simulink model "MPC_RL_H2DF"  (R2023a)
settings: Solver=FixedStepAuto  StartTime=0.0  StopTime=inf  FixedStep=Ts  RelTol=1e-3
model workspace (MAT data in the model file):
  enable_IMEP_noise = 100
  enable_IMEP_offset = 1
values from neighbouring files (symbols this model uses):
  C2C_NMPC = init_C2C_NMPC_H2DF(C2C_NMPC.expdata)    [init_H2DFRL_GRU.m]
  LowerLimit = ([0.17e-3;350;-5;1e-3] - C2C_NMPC.Normalization.controls.mean)./(C2C_NMPC.Normalization.controls.std)    [init_H2DFRL_GRU.m]
  Ts = 0.08    [init_H2DFRL_GRU.m]
  UpperLimit = ([0.5e-3;900;2;5.5e-3] - C2C_NMPC.Normalization.controls.mean)./(C2C_NMPC.Normalization.controls.std)    [init_H2DFRL_GRU.m]
undefined symbols (not defined in the file or in its folder): CA50_offset, DiscIntNeverNeededParam, enable_CA50_noise, enable_CA50_offset, IMEP_offset
libraries: simulink x15, matrix_library x6, dspsigattribs x2, slctrlblks x2, statsLibrary x1, rllib x1
(part 4 of 4)

== system MPC_RL_H2DF/Engine Model2/C2C_NMPC_n2/constraints/Normalizing data ==
  physical_data : Inport
  Constant1 : Constant  Value=C2C_NMPC.Normalization.controls.mean(2)
  Constant2 : Constant  Value=C2C_NMPC.Normalization.controls.mean(3)
  Constant3 : Constant  Value=C2C_NMPC.Normalization.controls.mean(1)
  Constant4 : Constant  Value=C2C_NMPC.Normalization.controls.mean(4)
  Gain1 : Gain  Gain=1/C2C_NMPC.Normalization.controls.std(2)
  Gain2 : Gain  Gain=1/C2C_NMPC.Normalization.controls.std(3)
  Gain3 : Gain  Gain=1/C2C_NMPC.Normalization.controls.std(4)
  Gain4 : Gain  Gain=1/C2C_NMPC.Normalization.controls.std(1)
  Mux : Mux
  Selector : Selector  IndexOptions=Index vector (dialog)  Indices=[2]  OutputSizes=1
  Selector1 : Selector  IndexOptions=Index vector (dialog)  Indices=[1]  OutputSizes=1
  Selector2 : Selector  IndexOptions=Index vector (dialog)  Indices=[3]  OutputSizes=1
  Selector3 : Selector  IndexOptions=Index vector (dialog)  Indices=[4]  OutputSizes=1
  Sum{1..4} (4 alike) : Sum  Inputs=|+-
  normalized_data : Outport
  wires:
  Constant3/1 -> Sum4/2
  Selector2/1 -> Sum3/1
  Constant2/1 -> Sum3/2
  Sum4/1 -> Gain4/1
  Sum3/1 -> Gain2/1
  Selector/1 -> Sum2/1
  Constant1/1 -> Sum2/2
  Sum2/1 -> Gain1/1
  Sum1/1 -> Gain3/1
  Constant4/1 -> Sum1/2
  Selector3/1 -> Sum1/1
  Selector1/1 -> Sum4/1
  Gain4/1 -> Mux/1
  Gain1/1 -> Mux/2
  Gain2/1 -> Mux/3
  Gain3/1 -> Mux/4
  Mux/1 -> normalized_data/1
  physical_data/1 -> Selector1/1, Selector/1, Selector3/1, Selector2/1

== system MPC_RL_H2DF/Engine Model2/C2C_NMPC_n2/constraints/Normalizing data1 ==
  physical_data : Inport
  Constant1 : Constant  Value=C2C_NMPC.Normalization.controls.mean(2)
  Constant2 : Constant  Value=C2C_NMPC.Normalization.controls.mean(3)
  Constant3 : Constant  Value=C2C_NMPC.Normalization.controls.mean(1)
  Constant4 : Constant  Value=C2C_NMPC.Normalization.controls.mean(4)
  Gain1 : Gain  Gain=1/C2C_NMPC.Normalization.controls.std(2)
  Gain2 : Gain  Gain=1/C2C_NMPC.Normalization.controls.std(3)
  Gain3 : Gain  Gain=1/C2C_NMPC.Normalization.controls.std(4)
  Gain4 : Gain  Gain=1/C2C_NMPC.Normalization.controls.std(1)
  Mux : Mux
  Selector : Selector  IndexOptions=Index vector (dialog)  Indices=[2]  OutputSizes=1
  Selector1 : Selector  IndexOptions=Index vector (dialog)  Indices=[1]  OutputSizes=1
  Selector2 : Selector  IndexOptions=Index vector (dialog)  Indices=[3]  OutputSizes=1
  Selector3 : Selector  IndexOptions=Index vector (dialog)  Indices=[4]  OutputSizes=1
  Sum{1..4} (4 alike) : Sum  Inputs=|+-
  normalized_data : Outport
  wires:
  Constant3/1 -> Sum4/2
  Selector2/1 -> Sum3/1
  Constant2/1 -> Sum3/2
  Sum4/1 -> Gain4/1
  Sum3/1 -> Gain2/1
  Selector/1 -> Sum2/1
  Constant1/1 -> Sum2/2
  Sum2/1 -> Gain1/1
  Sum1/1 -> Gain3/1
  Constant4/1 -> Sum1/2
  Selector3/1 -> Sum1/1
  Selector1/1 -> Sum4/1
  Gain4/1 -> Mux/1
  Gain1/1 -> Mux/2
  Gain2/1 -> Mux/3
  Gain3/1 -> Mux/4
  Mux/1 -> normalized_data/1
  physical_data/1 -> Selector1/1, Selector/1, Selector3/1, Selector2/1

== system MPC_RL_H2DF/Engine Model2/C2C_NMPC_n2/constraints/Subsystem ==
  In : Inport
  Constant : Constant  Value=C2C_NMPC.Normalization.outputs.mean(1)
  Constant1 : Constant  Value=C2C_NMPC.Normalization.outputs.mean(2)
  Constant2 : Constant  Value=C2C_NMPC.Normalization.outputs.mean(3)
  Constant3 : Constant  Value=C2C_NMPC.Normalization.outputs.mean(4)
  Demux : Demux
  Gain : Gain  Gain=1/C2C_NMPC.Normalization.outputs.std(1)
  Gain1 : Gain  Gain=1/C2C_NMPC.Normalization.outputs.std(2)
  Gain2 : Gain  Gain=1/C2C_NMPC.Normalization.outputs.std(3)
  Gain3 : Gain  Gain=1/C2C_NMPC.Normalization.outputs.std(4)
  Mux : Mux
  Sum{1..3,5} (4 alike) : Sum  Inputs=|+-
  value : Outport
  wires:
  Constant/1 -> Sum5/2
  Constant1/1 -> Sum1/2
  Sum1/1 -> Gain1/1
  Demux/3 -> Sum2/1
  Sum2/1 -> Gain2/1
  Constant2/1 -> Sum2/2
  Gain/1 -> Mux/1
  Sum3/1 -> Gain3/1
  Constant3/1 -> Sum3/2
  Sum5/1 -> Gain/1
  Demux/1 -> Sum5/1
  Gain2/1 -> Mux/3
  Gain3/1 -> Mux/4
  Gain1/1 -> Mux/2
  Demux/2 -> Sum1/1
  Demux/4 -> Sum3/1
  In/1 -> Demux/1
  Mux/1 -> value/1

== system MPC_RL_H2DF/Engine Model2/C2C_NMPC_n2/constraints/Subsystem1 ==
  In : Inport
  Constant : Constant  Value=C2C_NMPC.Normalization.outputs.mean(1)
  Constant1 : Constant  Value=C2C_NMPC.Normalization.outputs.mean(2)
  Constant2 : Constant  Value=C2C_NMPC.Normalization.outputs.mean(3)
  Constant3 : Constant  Value=C2C_NMPC.Normalization.outputs.mean(4)
  Demux : Demux
  Gain : Gain  Gain=1/C2C_NMPC.Normalization.outputs.std(1)
  Gain1 : Gain  Gain=1/C2C_NMPC.Normalization.outputs.std(2)
  Gain2 : Gain  Gain=1/C2C_NMPC.Normalization.outputs.std(3)
  Gain3 : Gain  Gain=1/C2C_NMPC.Normalization.outputs.std(4)
  Mux : Mux
  Sum{1..3,5} (4 alike) : Sum  Inputs=|+-
  ubh_e : Outport
  wires:
  Mux/1 -> ubh_e/1
  In/1 -> Demux/1
  Demux/4 -> Sum3/1
  Demux/2 -> Sum1/1
  Gain1/1 -> Mux/2
  Gain3/1 -> Mux/4
  Gain2/1 -> Mux/3
  Demux/1 -> Sum5/1
  Sum5/1 -> Gain/1
  Constant3/1 -> Sum3/2
  Sum3/1 -> Gain3/1
  Gain/1 -> Mux/1
  Constant2/1 -> Sum2/2
  Sum2/1 -> Gain2/1
  Demux/3 -> Sum2/1
  Sum1/1 -> Gain1/1
  Constant1/1 -> Sum1/2
  Constant/1 -> Sum5/2

== system MPC_RL_H2DF/Engine Model2/C2C_NMPC_n2/constraints/Subsystem2 ==
  In : Inport
  Demux : Demux
  Gain : Gain  Gain=1/C2C_NMPC.Normalization.controls.std(1)
  Gain1 : Gain  Gain=1/C2C_NMPC.Normalization.controls.std(2)
  Gain2 : Gain  Gain=1/C2C_NMPC.Normalization.controls.std(3)
  Gain3 : Gain  Gain=1/C2C_NMPC.Normalization.controls.std(4)
  Mux : Mux
  Out : Outport
  wires:
  Gain/1 -> Mux/1
  Gain2/1 -> Mux/3
  Gain1/1 -> Mux/2
  In/1 -> Demux/1
  Mux/1 -> Out/1
  Demux/1 -> Gain/1
  Demux/2 -> Gain1/1
  Demux/3 -> Gain2/1
  Demux/4 -> Gain3/1
  Gain3/1 -> Mux/4

== system MPC_RL_H2DF/Engine Model2/C2C_NMPC_n2/constraints/Subsystem3 ==
  In : Inport
  Demux : Demux
  Gain : Gain  Gain=1/C2C_NMPC.Normalization.controls.std(1)
  Gain1 : Gain  Gain=1/C2C_NMPC.Normalization.controls.std(2)
  Gain2 : Gain  Gain=1/C2C_NMPC.Normalization.controls.std(3)
  Gain3 : Gain  Gain=1/C2C_NMPC.Normalization.controls.std(4)
  Mux : Mux
  Out : Outport
  wires:
  Gain/1 -> Mux/1
  Gain2/1 -> Mux/3
  Gain1/1 -> Mux/2
  In/1 -> Demux/1
  Mux/1 -> Out/1
  Demux/1 -> Gain/1
  Demux/2 -> Gain1/1
  Demux/3 -> Gain2/1
  Demux/4 -> Gain3/1
  Gain3/1 -> Mux/4

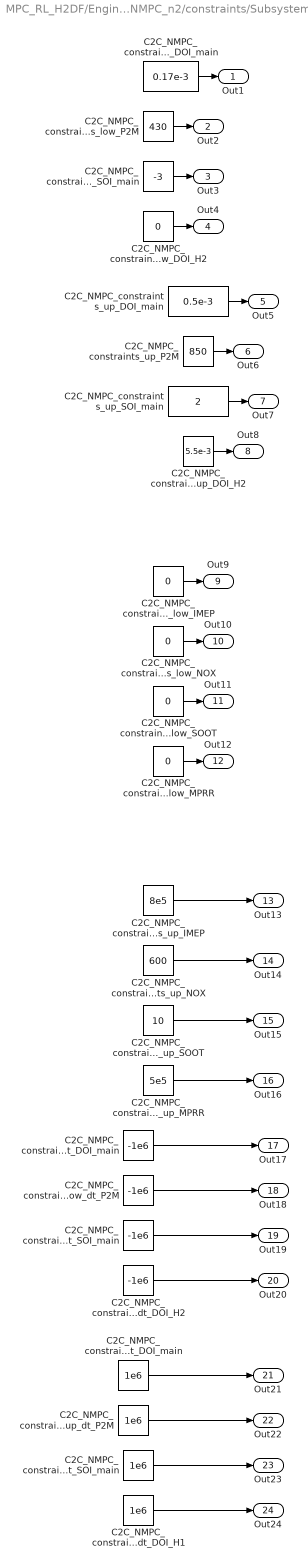
== system MPC_RL_H2DF/Engine Model2/C2C_NMPC_n2/constraints/Subsystem4 ==
  C2C_NMPC_constraints_low_DOI_H2 : Constant  Value=0
  C2C_NMPC_constraints_low_DOI_main : Constant  Value=0.17e-3
  C2C_NMPC_constraints_low_IMEP : Constant  Value=0
  C2C_NMPC_constraints_low_MPRR : Constant  Value=0
  C2C_NMPC_constraints_low_NOX : Constant  Value=0
  C2C_NMPC_constraints_low_P2M : Constant  Value=430
  C2C_NMPC_constraints_low_SOI_main : Constant  Value=-3
  C2C_NMPC_constraints_low_SOOT : Constant  Value=0
  C2C_NMPC_constraints_low_dt_DOI_H2 : Constant  Value=-1e6
  C2C_NMPC_constraints_low_dt_DOI_main : Constant  Value=-1e6
  C2C_NMPC_constraints_low_dt_P2M : Constant  Value=-1e6
  C2C_NMPC_constraints_low_dt_SOI_main : Constant  Value=-1e6
  C2C_NMPC_constraints_up_DOI_H2 : Constant  Value=5.5e-3
  C2C_NMPC_constraints_up_DOI_main : Constant  Value=0.5e-3
  C2C_NMPC_constraints_up_IMEP : Constant  Value=8e5
  C2C_NMPC_constraints_up_MPRR : Constant  Value=5e5
  C2C_NMPC_constraints_up_NOX : Constant  Value=600
  C2C_NMPC_constraints_up_P2M : Constant  Value=850
  C2C_NMPC_constraints_up_SOI_main : Constant  Value=2
  C2C_NMPC_constraints_up_SOOT : Constant  Value=10
  C2C_NMPC_constraints_up_dt_DOI_H1 : Constant  Value=1e6
  C2C_NMPC_constraints_up_dt_DOI_main : Constant  Value=1e6
  C2C_NMPC_constraints_up_dt_P2M : Constant  Value=1e6
  C2C_NMPC_constraints_up_dt_SOI_main : Constant  Value=1e6
  Out1 : Outport
  Out2 : Outport  Port=2
  Out3 : Outport  Port=3
  Out4 : Outport  Port=4
  Out5 : Outport  Port=5
  Out6 : Outport  Port=6
  Out7 : Outport  Port=7
  Out8 : Outport  Port=8
  Out9 : Outport  Port=9
  Out10 : Outport  Port=10
  Out11 : Outport  Port=11
  Out12 : Outport  Port=12
  Out13 : Outport  Port=13
  Out14 : Outport  Port=14
  Out15 : Outport  Port=15
  Out16 : Outport  Port=16
  Out17 : Outport  Port=17
  Out18 : Outport  Port=18
  Out19 : Outport  Port=19
  Out20 : Outport  Port=20
  Out21 : Outport  Port=21
  Out22 : Outport  Port=22
  Out23 : Outport  Port=23
  Out24 : Outport  Port=24
  wires:
  C2C_NMPC_constraints_low_dt_DOI_H2/1 -> Out20/1
  C2C_NMPC_constraints_low_dt_P2M/1 -> Out18/1
  C2C_NMPC_constraints_up_dt_SOI_main/1 -> Out23/1
  C2C_NMPC_constraints_up_dt_DOI_H1/1 -> Out24/1
  C2C_NMPC_constraints_up_DOI_H2/1 -> Out8/1
  C2C_NMPC_constraints_low_dt_DOI_main/1 -> Out17/1
  C2C_NMPC_constraints_low_dt_SOI_main/1 -> Out19/1
  C2C_NMPC_constraints_up_SOOT/1 -> Out15/1
  C2C_NMPC_constraints_up_MPRR/1 -> Out16/1
  C2C_NMPC_constraints_up_NOX/1 -> Out14/1
  C2C_NMPC_constraints_up_IMEP/1 -> Out13/1
  C2C_NMPC_constraints_up_dt_P2M/1 -> Out22/1
  C2C_NMPC_constraints_low_SOI_main/1 -> Out3/1
  C2C_NMPC_constraints_up_dt_DOI_main/1 -> Out21/1
  C2C_NMPC_constraints_low_SOOT/1 -> Out11/1
  C2C_NMPC_constraints_low_DOI_H2/1 -> Out4/1
  C2C_NMPC_constraints_up_P2M/1 -> Out6/1
  C2C_NMPC_constraints_low_P2M/1 -> Out2/1
  C2C_NMPC_constraints_low_DOI_main/1 -> Out1/1
  C2C_NMPC_constraints_low_MPRR/1 -> Out12/1
  C2C_NMPC_constraints_up_SOI_main/1 -> Out7/1
  C2C_NMPC_constraints_up_DOI_main/1 -> Out5/1
  C2C_NMPC_constraints_low_IMEP/1 -> Out9/1
  C2C_NMPC_constraints_low_NOX/1 -> Out10/1

== system MPC_RL_H2DF/Engine Model2/C2C_NMPC_n2/cost_function_weights/Normalize 0 to 1 ==
  In1 : Inport
  Demux : Demux
  Divide{,1..3} (4 alike) : Product  Inputs=*/
  Mux : Mux
  Sum : Sum  Inputs=|++++
  Out1 : Outport
  wires:
  In1/1 -> Demux/1
  Demux/1 -> Sum/1, Divide/1
  Demux/2 -> Divide1/1, Sum/2
  Demux/3 -> Divide2/1, Sum/3
  Demux/4 -> Divide3/1, Sum/4
  Sum/1 -> Divide/2, Divide1/2, Divide2/2, Divide3/2
  Divide3/1 -> Mux/4
  Divide2/1 -> Mux/3
  Divide1/1 -> Mux/2
  Divide/1 -> Mux/1
  Mux/1 -> Out1/1

== system MPC_RL_H2DF/Engine Model2/offset_and_noise/CA50_generation/denormalizing_CA50 ==
  CA50_in : Inport
  Constant : Constant  Value=C2C_NMPC.Normalization.outputs.mean(4)
  Gain : Gain  Gain=C2C_NMPC.Normalization.outputs.std(4)
  Sum5 : Sum  Inputs=|++
  CA50 : Outport
  wires:
  CA50_in/1 -> Gain/1
  Gain/1 -> Sum5/1
  Constant/1 -> Sum5/2
  Sum5/1 -> CA50/1

== system MPC_RL_H2DF/Engine Model2/offset_and_noise/CA50_generation/normalizing_CA50 ==
  CA50 : Inport
  Constant : Constant  Value=C2C_NMPC.Normalization.outputs.mean(4)
  Gain : Gain  Gain=1/C2C_NMPC.Normalization.outputs.std(4)
  Sum5 : Sum  Inputs=|+-
  CA50_out : Outport
  wires:
  CA50/1 -> Sum5/1
  Constant/1 -> Sum5/2
  Gain/1 -> CA50_out/1
  Sum5/1 -> Gain/1

== system MPC_RL_H2DF/Engine Model2/offset_and_noise/IMEP_generation/denormalizing_IMEP ==
  IMEP_in : Inport
  Constant : Constant  Value=C2C_NMPC.Normalization.outputs.mean(1)
  Gain : Gain  Gain=C2C_NMPC.Normalization.outputs.std(1)
  Sum5 : Sum  Inputs=|++
  IMEP : Outport
  wires:
  IMEP_in/1 -> Gain/1
  Gain/1 -> Sum5/1
  Constant/1 -> Sum5/2
  Sum5/1 -> IMEP/1

== system MPC_RL_H2DF/Engine Model2/offset_and_noise/IMEP_generation/normalizing_IMEP ==
  IMEP : Inport
  Constant : Constant  Value=C2C_NMPC.Normalization.outputs.mean(1)
  Gain : Gain  Gain=1/C2C_NMPC.Normalization.outputs.std(1)
  Sum5 : Sum  Inputs=|+-
  IMEP_out : Outport
  wires:
  IMEP/1 -> Sum5/1
  Constant/1 -> Sum5/2
  Gain/1 -> IMEP_out/1
  Sum5/1 -> Gain/1

== system MPC_RL_H2DF/Engine Model2/offset_and_noise1/IMEP_generation/denormalizing_IMEP ==
  IMEP_in : Inport
  Constant : Constant  Value=C2C_NMPC.Normalization.outputs.mean(1)
  Gain : Gain  Gain=C2C_NMPC.Normalization.outputs.std(1)
  Sum5 : Sum  Inputs=|++
  IMEP : Outport
  wires:
  IMEP_in/1 -> Gain/1
  Gain/1 -> Sum5/1
  Constant/1 -> Sum5/2
  Sum5/1 -> IMEP/1

== system MPC_RL_H2DF/Engine Model2/offset_and_noise1/IMEP_generation/normalizing_IMEP ==
  IMEP : Inport
  Constant : Constant  Value=C2C_NMPC.Normalization.outputs.mean(1)
  Gain : Gain  Gain=1/C2C_NMPC.Normalization.outputs.std(1)
  Sum5 : Sum  Inputs=|+-
  IMEP_out : Outport
  wires:
  IMEP/1 -> Sum5/1
  Constant/1 -> Sum5/2
  Gain/1 -> IMEP_out/1
  Sum5/1 -> Gain/1

== system MPC_RL_H2DF/Engine Model2/offset_and_noise2/IMEP_generation/denormalizing_IMEP ==
  IMEP_in : Inport
  Constant : Constant  Value=C2C_NMPC.Normalization.outputs.mean(1)
  Gain : Gain  Gain=C2C_NMPC.Normalization.outputs.std(1)
  Sum5 : Sum  Inputs=|++
  IMEP : Outport
  wires:
  IMEP_in/1 -> Gain/1
  Gain/1 -> Sum5/1
  Constant/1 -> Sum5/2
  Sum5/1 -> IMEP/1

== system MPC_RL_H2DF/Engine Model2/offset_and_noise2/IMEP_generation/normalizing_IMEP ==
  IMEP : Inport
  Constant : Constant  Value=C2C_NMPC.Normalization.outputs.mean(1)
  Gain : Gain  Gain=1/C2C_NMPC.Normalization.outputs.std(1)
  Sum5 : Sum  Inputs=|+-
  IMEP_out : Outport
  wires:
  IMEP/1 -> Sum5/1
  Constant/1 -> Sum5/2
  Gain/1 -> IMEP_out/1
  Sum5/1 -> Gain/1

== system MPC_RL_H2DF/Engine Model2/offset_and_noise3/IMEP_generation/denormalizing_IMEP ==
  IMEP_in : Inport
  Constant : Constant  Value=C2C_NMPC.Normalization.outputs.mean(1)
  Gain : Gain  Gain=C2C_NMPC.Normalization.outputs.std(1)
  Sum5 : Sum  Inputs=|++
  IMEP : Outport
  wires:
  IMEP_in/1 -> Gain/1
  Gain/1 -> Sum5/1
  Constant/1 -> Sum5/2
  Sum5/1 -> IMEP/1

== system MPC_RL_H2DF/Engine Model2/offset_and_noise3/IMEP_generation/normalizing_IMEP ==
  IMEP : Inport
  Constant : Constant  Value=C2C_NMPC.Normalization.outputs.mean(1)
  Gain : Gain  Gain=1/C2C_NMPC.Normalization.outputs.std(1)
  Sum5 : Sum  Inputs=|+-
  IMEP_out : Outport
  wires:
  IMEP/1 -> Sum5/1
  Constant/1 -> Sum5/2
  Gain/1 -> IMEP_out/1
  Sum5/1 -> Gain/1

== system MPC_RL_H2DF/Signal Processing/calculate reward/Subsystem/ControlError ==
  ReferenceControls : Inport
  Controls : Inport  Port=2
  Demux1 : Demux
  Demux2 : Demux
  Mux : Mux
  Subtract{,1..3} (4 alike) : Sum  Inputs=+-
  ControlError : Outport
  wires:
  Demux2/4 -> Subtract3/2
  Demux1/2 -> Subtract1/1
  Demux1/1 -> Subtract/1
  Demux2/2 -> Subtract1/2
  Demux2/3 -> Subtract2/2
  Controls/1 -> Demux2/1
  Demux1/3 -> Subtract2/1
  Demux1/4 -> Subtract3/1
  Demux2/1 -> Subtract/2
  Mux/1 -> ControlError/1
  Subtract/1 -> Mux/1
  Subtract1/1 -> Mux/2
  Subtract2/1 -> Mux/3
  Subtract3/1 -> Mux/4
  ReferenceControls/1 -> Demux1/1

== system MPC_RL_H2DF/Signal Processing/calculate reward/Subsystem/Staging ==
  Output : Inport
  Reference_Output : Inport  Port=2
  Abs4 : Abs  SaturateOnIntegerOverflow=off
  Add : Sum  Inputs=++++
  Constant : Constant  Value=100000
  Constant1 : Constant  Value=10000
  Constant2 : Constant  Value=1000
  Constant3 : Constant  Value=100
  Demux : Demux
  Demux6 : Demux
  Display{,1..4} (5 alike) : Display
  Gain1 : Gain  Gain=-25
  Gain3 : Gain  Gain=-100
  Gain4 : Gain  Gain=-500
  Gain5 : Gain  Gain=-5000
  Gain6 : Gain  Gain=0.1
  Relational Operator{,1..3} (4 alike) : RelationalOperator  Operator=<=  OutDataTypeStr=boolean  RndMeth=Simplest  InputSameDT=off
  Scope : Scope  NumInputPorts=3
  Subsystem : Subsystem
  Subsystem1 : Subsystem
  Sum6 : Sum  Inputs=+-
  Out1 : Outport
  wires:
  Reference_Output/1 -> Demux/1
  Gain5/1 -> Add/4
  Gain4/1 -> Add/3
  Relational Operator1/1 -> Gain3/1
  Demux6/1 -> Subsystem/1(IMEP_norm1)
  Gain3/1 -> Add/2
  Relational Operator3/1 -> Gain5/1
  Demux/1 -> Subsystem1/1(IMEP_norm1)
  Output/1 -> Demux6/1
  Relational Operator2/1 -> Gain4/1
  Add/1 -> Display2/1, Gain6/1
  Relational Operator/1 -> Display/1, Gain1/1
  Abs4/1 -> Display3/1, Relational Operator/1, Relational Operator1/1, Relational Operator2/1, Relational Operator3/1
  Sum6/1 -> Abs4/1
  Gain1/1 -> Display1/1, Add/1
  Constant3/1 -> Relational Operator3/2
  Constant2/1 -> Relational Operator2/2
  Constant1/1 -> Relational Operator1/2
  Constant/1 -> Display4/1, Relational Operator/2
  Gain6/1 -> Scope/3, Out1/1
  Subsystem/1(IMEP1) -> Scope/2, Sum6/2
  Subsystem1/1(IMEP1) -> Sum6/1, Scope/1

== system MPC_RL_H2DF/Signal Processing/calculate reward/Subsystem/Subsystem ==
  Data Store Read18 : DataStoreRead  DataStoreName=C2C_NMPC_constraints_up_SOOT  IndexOptions=Index vector (dialog)  Indices=1  OutputSizes=1
  Data Store Read19 : DataStoreRead  DataStoreName=C2C_NMPC_constraints_low_NOX  IndexOptions=Index vector (dialog)  Indices=1  OutputSizes=1
  Data Store Read20 : DataStoreRead  DataStoreName=C2C_NMPC_constraints_low_SOOT  IndexOptions=Index vector (dialog)  Indices=1  OutputSizes=1
  Data Store Read21 : DataStoreRead  DataStoreName=C2C_NMPC_constraints_low_MPRR  IndexOptions=Index vector (dialog)  Indices=1  OutputSizes=1
  Data Store Read22 : DataStoreRead  DataStoreName=C2C_NMPC_constraints_up_MPRR  IndexOptions=Index vector (dialog)  Indices=1  OutputSizes=1
  Data Store Read5 : DataStoreRead  DataStoreName=C2C_NMPC_constraints_low_IMEP  IndexOptions=Index vector (dialog)  Indices=1  OutputSizes=1
  Data Store Read6 : DataStoreRead  DataStoreName=C2C_NMPC_constraints_up_IMEP  IndexOptions=Index vector (dialog)  Indices=1  OutputSizes=1
  Data Store Read7 : DataStoreRead  DataStoreName=C2C_NMPC_constraints_up_NOX  IndexOptions=Index vector (dialog)  Indices=1  OutputSizes=1
  Demux : Demux
  Demux5 : Demux
  Mux : Mux
  Mux1 : Mux
  Normalize Physical Controls and Outputs2 : Subsystem
  Normalize Physical Controls and Outputs3 : Subsystem
  Terminator : Terminator
  Terminator1 : Terminator
  Out1 : Outport
  Out2 : Outport  Port=2
  Out3 : Outport  Port=3
  Out4 : Outport  Port=4
  Out5 : Outport  Port=5
  Out6 : Outport  Port=6
  Out7 : Outport  Port=7
  Out8 : Outport  Port=8
  wires:
  Normalize Physical Controls and Outputs2/1("NormalisedControls ") -> Terminator/1
  Data Store Read6/1 -> Mux/1
  Normalize Physical Controls and Outputs3/2(NormalisedOutputs) -> Demux5/1
  Data Store Read5/1 -> Mux1/1
  Demux5/3 -> Out6/1
  Data Store Read18/1 -> Mux/3
  Normalize Physical Controls and Outputs2/2(NormalisedOutputs) -> Demux/1
  Data Store Read21/1 -> Mux1/4
  Mux1/1 -> Normalize Physical Controls and Outputs3/2("ouputs ")
  Demux/3 -> Out5/1
  Data Store Read20/1 -> Mux1/3
  Normalize Physical Controls and Outputs3/1("NormalisedControls ") -> Terminator1/1
  Data Store Read19/1 -> Mux1/2
  Data Store Read22/1 -> Mux/4
  Demux/1 -> Out1/1
  Data Store Read7/1 -> Mux/2
  Mux/1 -> Normalize Physical Controls and Outputs2/2("ouputs ")
  Demux/2 -> Out3/1
  Demux5/4 -> Out8/1
  Demux5/2 -> Out4/1
  Demux5/1 -> Out2/1
  Demux/4 -> Out7/1

== system MPC_RL_H2DF/Signal Processing/calculate reward/Subsystem/TrackingError ==
  Outputs : Inport
  ReferenceOutputs : Inport  Port=2
  Demux1 : Demux
  Demux2 : Demux
  Mux : Mux
  Subtract{,1..3} (4 alike) : Sum  Inputs=+-
  TrackingError : Outport
  wires:
  Demux2/4 -> Subtract3/2
  Demux1/2 -> Subtract1/1
  Demux1/1 -> Subtract/1
  Demux2/2 -> Subtract1/2
  Demux2/3 -> Subtract2/2
  Outputs/1 -> Demux2/1
  Demux1/3 -> Subtract2/1
  Demux1/4 -> Subtract3/1
  Demux2/1 -> Subtract/2
  Mux/1 -> TrackingError/1
  Subtract/1 -> Mux/1
  Subtract1/1 -> Mux/2
  Subtract2/1 -> Mux/3
  Subtract3/1 -> Mux/4
  ReferenceOutputs/1 -> Demux1/1

== system MPC_RL_H2DF/Signal Processing/calculate reward/Subsystem/Staging/Subsystem ==
  IMEP_norm1 : Inport
  Constant4 : Constant  Value=C2C_NMPC.Normalization.outputs.mean(1)
  Gain2 : Gain  Gain=C2C_NMPC.Normalization.outputs.std(1)
  Sum4 : Sum  Inputs=|++
  IMEP1 : Outport
  wires:
  Sum4/1 -> IMEP1/1
  Constant4/1 -> Sum4/2
  Gain2/1 -> Sum4/1
  IMEP_norm1/1 -> Gain2/1

== system MPC_RL_H2DF/Signal Processing/calculate reward/Subsystem/Staging/Subsystem1 ==
  IMEP_norm1 : Inport
  Constant4 : Constant  Value=C2C_NMPC.Normalization.outputs.mean(1)
  Gain2 : Gain  Gain=C2C_NMPC.Normalization.outputs.std(1)
  Sum4 : Sum  Inputs=|++
  IMEP1 : Outport
  wires:
  Sum4/1 -> IMEP1/1
  Constant4/1 -> Sum4/2
  Gain2/1 -> Sum4/1
  IMEP_norm1/1 -> Gain2/1

== system MPC_RL_H2DF/Signal Processing/calculate reward/Subsystem/Subsystem/Normalize Physical Controls and Outputs2 ==
  controls : Inport
  "ouputs " : Inport  Port=2
  Constant : Constant  Value=C2C_NMPC.Normalization.outputs.mean(1)
  Constant1 : Constant  Value=C2C_NMPC.Normalization.outputs.mean(2)
  Constant10 : Constant  Value=C2C_NMPC.Normalization.controls.mean(2)
  Constant11 : Constant  Value=C2C_NMPC.Normalization.controls.mean(3)
  Constant12 : Constant  Value=C2C_NMPC.Normalization.controls.mean(4)
  Constant2 : Constant  Value=C2C_NMPC.Normalization.outputs.mean(3)
  Constant3 : Constant  Value=C2C_NMPC.Normalization.outputs.mean(4)
  Constant9 : Constant  Value=C2C_NMPC.Normalization.controls.mean(1)
  Demux : Demux
  Demux1 : Demux
  Gain : Gain  Gain=1/C2C_NMPC.Normalization.outputs.std(1)
  Gain1 : Gain  Gain=1/C2C_NMPC.Normalization.outputs.std(2)
  Gain2 : Gain  Gain=1/C2C_NMPC.Normalization.outputs.std(3)
  Gain3 : Gain  Gain=1/C2C_NMPC.Normalization.outputs.std(4)
  Gain4 : Gain  Gain=1/C2C_NMPC.Normalization.controls.std(1)
  Gain5 : Gain  Gain=1/C2C_NMPC.Normalization.controls.std(2)
  Gain6 : Gain  Gain=1/C2C_NMPC.Normalization.controls.std(3)
  Gain7 : Gain  Gain=1/C2C_NMPC.Normalization.controls.std(4)
  Mux1 : Mux
  Mux2 : Mux
  Sum{1,6..12} (8 alike) : Sum  Inputs=|+-
  "NormalisedControls " : Outport
  NormalisedOutputs : Outport  Port=2
  wires:
  Constant2/1 -> Sum6/2
  Gain7/1 -> Mux1/4
  Gain5/1 -> Mux1/2
  Constant12/1 -> Sum12/2
  Constant11/1 -> Sum11/2
  Gain4/1 -> Mux1/1
  Demux/1 -> Sum8/1
  Demux1/2 -> Sum1/1
  Constant/1 -> Sum9/2
  Sum11/1 -> Gain6/1
  Demux/4 -> Sum12/1
  Gain6/1 -> Mux1/3
  Constant1/1 -> Sum1/2
  Demux1/4 -> Sum7/1
  Demux1/3 -> Sum6/1
  Sum6/1 -> Gain2/1
  Sum9/1 -> Gain/1
  Sum10/1 -> Gain5/1
  Mux1/1 -> "NormalisedControls "/1
  Sum8/1 -> Gain4/1
  Sum12/1 -> Gain7/1
  Constant9/1 -> Sum8/2
  Demux/2 -> Sum10/1
  Constant10/1 -> Sum10/2
  Constant3/1 -> Sum7/2
  Sum1/1 -> Gain1/1
  Demux/3 -> Sum11/1
  Sum7/1 -> Gain3/1
  controls/1 -> Demux/1
  "ouputs "/1 -> Demux1/1
  Demux1/1 -> Sum9/1
  Gain1/1 -> Mux2/2
  Gain/1 -> Mux2/1
  Gain2/1 -> Mux2/3
  Gain3/1 -> Mux2/4
  Mux2/1 -> NormalisedOutputs/1

== system MPC_RL_H2DF/Signal Processing/calculate reward/Subsystem/Subsystem/Normalize Physical Controls and Outputs3 ==
  controls : Inport
  "ouputs " : Inport  Port=2
  Constant : Constant  Value=C2C_NMPC.Normalization.outputs.mean(1)
  Constant1 : Constant  Value=C2C_NMPC.Normalization.outputs.mean(2)
  Constant10 : Constant  Value=C2C_NMPC.Normalization.controls.mean(2)
  Constant11 : Constant  Value=C2C_NMPC.Normalization.controls.mean(3)
  Constant12 : Constant  Value=C2C_NMPC.Normalization.controls.mean(4)
  Constant2 : Constant  Value=C2C_NMPC.Normalization.outputs.mean(3)
  Constant3 : Constant  Value=C2C_NMPC.Normalization.outputs.mean(4)
  Constant9 : Constant  Value=C2C_NMPC.Normalization.controls.mean(1)
  Demux : Demux
  Demux1 : Demux
  Gain : Gain  Gain=1/C2C_NMPC.Normalization.outputs.std(1)
  Gain1 : Gain  Gain=1/C2C_NMPC.Normalization.outputs.std(2)
  Gain2 : Gain  Gain=1/C2C_NMPC.Normalization.outputs.std(3)
  Gain3 : Gain  Gain=1/C2C_NMPC.Normalization.outputs.std(4)
  Gain4 : Gain  Gain=1/C2C_NMPC.Normalization.controls.std(1)
  Gain5 : Gain  Gain=1/C2C_NMPC.Normalization.controls.std(2)
  Gain6 : Gain  Gain=1/C2C_NMPC.Normalization.controls.std(3)
  Gain7 : Gain  Gain=1/C2C_NMPC.Normalization.controls.std(4)
  Mux1 : Mux
  Mux2 : Mux
  Sum{1,6..12} (8 alike) : Sum  Inputs=|+-
  "NormalisedControls " : Outport
  NormalisedOutputs : Outport  Port=2
  wires:
  Constant2/1 -> Sum6/2
  Gain7/1 -> Mux1/4
  Gain5/1 -> Mux1/2
  Constant12/1 -> Sum12/2
  Constant11/1 -> Sum11/2
  Gain4/1 -> Mux1/1
  Demux/1 -> Sum8/1
  Demux1/2 -> Sum1/1
  Constant/1 -> Sum9/2
  Sum11/1 -> Gain6/1
  Demux/4 -> Sum12/1
  Gain6/1 -> Mux1/3
  Constant1/1 -> Sum1/2
  Demux1/4 -> Sum7/1
  Demux1/3 -> Sum6/1
  Sum6/1 -> Gain2/1
  Sum9/1 -> Gain/1
  Sum10/1 -> Gain5/1
  Mux1/1 -> "NormalisedControls "/1
  Sum8/1 -> Gain4/1
  Sum12/1 -> Gain7/1
  Constant9/1 -> Sum8/2
  Demux/2 -> Sum10/1
  Constant10/1 -> Sum10/2
  Constant3/1 -> Sum7/2
  Sum1/1 -> Gain1/1
  Demux/3 -> Sum11/1
  Sum7/1 -> Gain3/1
  controls/1 -> Demux/1
  "ouputs "/1 -> Demux1/1
  Demux1/1 -> Sum9/1
  Gain1/1 -> Mux2/2
  Gain/1 -> Mux2/1
  Gain2/1 -> Mux2/3
  Gain3/1 -> Mux2/4
  Mux2/1 -> NormalisedOutputs/1

== matlab function MPC_RL_H2DF/Engine Model2/C2C_NMPC_n1/constraints/MATLAB Function2 ==
  data: value input; vector output; length input; init_vector input
function vector = fcn(value, length, init_vector)
init_vector(1:(size(value,1)*length)) = repmat(value, length, 1);
vector = init_vector;

== matlab function MPC_RL_H2DF/Engine Model2/C2C_NMPC_n1/constraints/MATLAB Function3 ==
  data: value input; vector output; length input; init_vector input
function vector = fcn(value, length, init_vector)
init_vector(1:(size(value,1)*length)) = repmat(value, length, 1);
vector = init_vector;

== matlab function MPC_RL_H2DF/Engine Model2/C2C_NMPC_n1/cost_function_weights/blkdiag Function ==
  data: u1 input; y output; u2 input; u3 input
 function y = fcn(u1,u2,u3)
y = reshape(blkdiag(u1, u2, u3),[],1);

== matlab function MPC_RL_H2DF/Engine Model2/C2C_NMPC_n1/cost_function_weights/blkdiag Function1 ==
  data: u1 input; y output; u2 input
function y = fcn(u1,u2)
y = reshape(blkdiag(u1, u2),[],1);

== matlab function MPC_RL_H2DF/Engine Model2/dyn_H2DF2/dyn_H2DF ==
  data: last_LSTM_states_MPC input; controls_MPC input; outputs_MPC output; last_outputs_MPC input; H2DF_Par parameter; LSTM_states_MPC output
 function [outputs_MPC, LSTM_states_MPC] = dyn_H2DF(last_LSTM_states_MPC, controls_MPC, last_outputs_MPC, H2DF_Par)

[outputs_MPC, LSTM_states_MPC] = dyn_H2DF_GRU(last_LSTM_states_MPC, [controls_MPC; last_outputs_MPC(1)], H2DF_Par);

== matlab function MPC_RL_H2DF/Engine Model2/dyn_H2DF_state_augmentation2/dyn_H2DF_state_augmentation ==
  data: last_LSTM_states_MPC input; LSTM_states output; controls_MPC input; last_outputs_MPC input; H2DF_Par parameter
function LSTM_states = dyn_H2DF_state_augmentation(last_LSTM_states_MPC, controls_MPC, last_outputs_MPC, H2DF_Par)

LSTM_states = dyn_H2DF_state_augmentation_GRU(last_LSTM_states_MPC,[controls_MPC; last_outputs_MPC(1)], H2DF_Par);

== matlab function MPC_RL_H2DF/Engine Model2/C2C_NMPC_n2/constraints/MATLAB Function ==
  data: value input; vector output; length input; init_vector input
function vector = fcn(value, length, init_vector)
init_vector(1:(size(value,1)*length)) = repmat(value, length, 1);
vector = init_vector;

== matlab function MPC_RL_H2DF/Engine Model2/C2C_NMPC_n2/constraints/MATLAB Function1 ==
  data: value input; vector output; length input; init_vector input
function vector = fcn(value, length, init_vector)
init_vector(1:(size(value,1)*length)) = repmat(value, length, 1);
vector = init_vector;

== matlab function MPC_RL_H2DF/Engine Model2/C2C_NMPC_n2/constraints/MATLAB Function2 ==
  data: value input; vector output; length input; init_vector input
function vector = fcn(value, length, init_vector)
init_vector(1:(size(value,1)*length)) = repmat(value, length, 1);
vector = init_vector;

== matlab function MPC_RL_H2DF/Engine Model2/C2C_NMPC_n2/constraints/MATLAB Function3 ==
  data: value input; vector output; length input; init_vector input
function vector = fcn(value, length, init_vector)
init_vector(1:(size(value,1)*length)) = repmat(value, length, 1);
vector = init_vector;

== matlab function MPC_RL_H2DF/Engine Model2/C2C_NMPC_n2/cost_function_weights/blkdiag Function ==
  data: u1 input; y output; u2 input; u3 input
 function y = fcn(u1,u2,u3)
y = reshape(blkdiag(u1, u2, u3),[],1);

== matlab function MPC_RL_H2DF/Engine Model2/C2C_NMPC_n2/cost_function_weights/blkdiag Function1 ==
  data: u1 input; y output; u2 input
function y = fcn(u1,u2)
y = reshape(blkdiag(u1, u2),[],1);

== matlab function MPC_RL_H2DF/Engine Model2/dyn_H2DF/dyn_H2DF ==
  data: last_LSTM_states input; controls input; outputs output; last_outputs input; H2DF_Par parameter; LSTM_states output
 function [outputs, LSTM_states] = dyn_H2DF(last_LSTM_states, controls, last_outputs, H2DF_Par)

[outputs, LSTM_states] = dyn_H2DF_GRU(last_LSTM_states, [controls; last_outputs(1)], H2DF_Par);

== matlab function MPC_RL_H2DF/Engine Model2/dyn_H2DF1/dyn_H2DF ==
  data: last_LSTM_states_MPC input; controls_MPC input; outputs_MPC output; last_outputs_MPC input; H2DF_Par parameter; LSTM_states_MPC output
 function [outputs_MPC, LSTM_states_MPC] = dyn_H2DF(last_LSTM_states_MPC, controls_MPC, last_outputs_MPC, H2DF_Par)

[outputs_MPC, LSTM_states_MPC] = dyn_H2DF_GRU(last_LSTM_states_MPC, [controls_MPC; last_outputs_MPC(1)], H2DF_Par);

== matlab function MPC_RL_H2DF/Engine Model2/dyn_H2DF_state_augmentation/dyn_H2DF_state_augmentation ==
  data: last_LSTM_states input; LSTM_states output; controls input; last_outputs input; H2DF_Par parameter
function LSTM_states = dyn_H2DF_state_augmentation(last_LSTM_states, controls, last_outputs, H2DF_Par)

LSTM_states = dyn_H2DF_state_augmentation_GRU(last_LSTM_states,[controls; last_outputs(1)], H2DF_Par);

== matlab function MPC_RL_H2DF/Engine Model2/reference1/ref_func ==
  data: ref_norm input; y_ref output; init_index input
  function y_ref = ref_func(ref_norm, init_index)

y_ref = ref_norm(:, init_index);

== matlab function MPC_RL_H2DF/Engine Model2/dyn_H2DF_state_augmentation1/dyn_H2DF_state_augmentation ==
  data: last_LSTM_states_MPC input; LSTM_states output; controls_MPC input; last_outputs_MPC input; H2DF_Par parameter
function LSTM_states = dyn_H2DF_state_augmentation(last_LSTM_states_MPC, controls_MPC, last_outputs_MPC, H2DF_Par)

LSTM_states = dyn_H2DF_state_augmentation_GRU(last_LSTM_states_MPC,[controls_MPC; last_outputs_MPC(1)], H2DF_Par);

== matlab function MPC_RL_H2DF/Engine Model2/C2C_NMPC_n1/constraints/MATLAB Function ==
  data: value input; vector output; length input; init_vector input
function vector = fcn(value, length, init_vector)
init_vector(1:(size(value,1)*length)) = repmat(value, length, 1);
vector = init_vector;

== matlab function MPC_RL_H2DF/Engine Model2/C2C_NMPC_n1/constraints/MATLAB Function1 ==
  data: value input; vector output; length input; init_vector input
function vector = fcn(value, length, init_vector)
init_vector(1:(size(value,1)*length)) = repmat(value, length, 1);
vector = init_vector;

== matlab function MPC_RL_H2DF/references/MATLAB Function ==
  data: t input; IMEP_ref output; rchange1 input; NOx_ref output; SOOT_ref output; MPRR_ref output; DOI_Main_ref output; P2M_ref output; SOI_ref output; DOI_H2_ref output; rchange2 input; rchange3 input; rchange4 input
function [IMEP_ref, NOx_ref, SOOT_ref, MPRR_ref, DOI_Main_ref, P2M_ref, SOI_ref, DOI_H2_ref] = fcn(t, rchange1,rchange2,rchange3,rchange4)
% IMEP_ref =5e5;
% NOx_ref =    66.8796;
% SOOT_ref= 0.2830;
% MPRR_ref= 17416;
% DOI_Main_ref =    1.7005e-04; 
% P2M_ref= 430;
% SOI_ref= -5.9815;
% DOI_H2_ref= 0.0017;

IMEP_ref = 5e5;
NOx_ref = 0;
SOOT_ref= 0;
MPRR_ref= 0;
DOI_Main_ref = 0; 
P2M_ref= 0;
SOI_ref= 0;
DOI_H2_ref= 0;

IMEP_ref = rchange1;
if t>1 && t<7.5
  IMEP_ref = rchange1; %[Outputs, Controls]
 
elseif t>=7.5 && t<15 
  IMEP_ref = rchange1*rchange2;

elseif t>=15  && t<25
  IMEP_ref = rchange1*rchange2*rchange3;

elseif t>=25  && t<30
  IMEP_ref = rchange1*rchange3;

elseif t>=30 && t<35
    IMEP_ref = (1-(t-30)/5)*rchange1*rchange3+((t-30)/5)*rchange1*rchange4; 

elseif t>35 && t<45
    IMEP_ref = rchange1*rchange4;

elseif t>=45 && t<60 
    IMEP_ref = (1-(t-45)/15)*rchange1*rchange4+((t-45)/15)*rchange1*rchange2*rchange3*rchange4;

elseif t>=60  && t<75
    IMEP_ref = rchange1*rchange2*rchange3*rchange4;

elseif t>=75 && t<100 
    IMEP_ref = (1-(t-75)/25)*rchange1*rchange2*rchange3*rchange4+((t-75)/25)*rchange1*rchange2*rchange4;
 
elseif t>=100
    IMEP_ref = rchange1*rchange2*rchange4;

end

if IMEP_ref<3e5
    IMEP_ref = 3e5;
elseif IMEP_ref > 8e5
    IMEP_ref = 8e5;
end

% 
% if t>4
%  IMEP_ref = 0.8*rchange; %[Outputs, Controls]
% end
% if t>5 
%     IMEP_ref = 0.6*rchange;
% end
% if t>6 
%     IMEP_ref = 1.4*rchange;
% end
% if t>7
%  IMEP_ref = rchange; %[Outputs, Controls]
% end
% if t>8 
%     IMEP_ref = 0.4*rchange;
% end
% if t>9 
%     IMEP_ref = 1.1*rchange;
% end
